simulink model "frequence_response_point3"  (R2019b)
settings: Solver=ode45  StartTime=0.0  StopTime=30  RelTol=1e-3  EnableMultiTasking=on
values from neighbouring files (symbols this model uses):
  C = [1 1 0 0;0 0 1 1]    [es1.m]
  phi = [0 0]    [es1.m]
  U = [1 -0.25]    [es1.m]
  w = [0 2]    [es1.m]
undefined symbols (not defined in the file or in its folder): A, B, D
settings Model: Creator=stefano  LastModifiedBy=Chiara
settings DataIOCC: LimitDataPoints=on  SaveFormat=Array  SignalLoggingSaveFormat=ModelDataLogs  ReturnWorkspaceOutputs=off
settings OptimizationCC: ExpressionDepthLimit=2147483647  LifeSpan=inf
settings DebuggingCC: UnderspecifiedInitializationDetection=Classic  MergeDetectMultiDrivingBlocksExec=none  SolverPrmCheckMsg=warning  FcnCallInpInsideContextMsg=warning  StateNameClashWarn=warning  SFUnexpectedBacktrackingDiag=warning  SFNoUnconditionalDefaultTransitionDiag=warning  SFExecutionAtInitializationDiag=none  ArithmeticOperatorsInVariantConditions=warning
settings HardwareCC: ProdBitPerPointer=32  ProdBitPerSizeT=32  ProdBitPerPtrDiffT=32  ProdLargestAtomicFloat=None  ProdIntDivRoundTo=Undefined  ProdEndianess=Unspecified  ProdWordSize=32  ProdHWDeviceType=32-bit Generic
settings ModelReferenceCC: PropagateSignalLabelsOutOfModel=off
settings SFSimCC: SimUseLocalCustomCode=off  CustomCodeUndefinedFunction=UseInterfaceOnly
settings RTWCC: RTWUseLocalCustomCode=off
settings CodeAppCC: StateflowObjectComments=on
settings GRTTargetCC: TargetLangStandard=C89/C90 (ANSI)  GeneratePreprocessorConditionals=Disable all  CombineOutputUpdateFcns=off  GRTInterface=on
settings ConfigComp: CovMetricSettings=dw  CovHtmlReporting=on  CovSaveCumulativeToWorkspaceVar=on  CovSaveSingleToWorkspaceVar=on  CovExternalEMLEnable=off

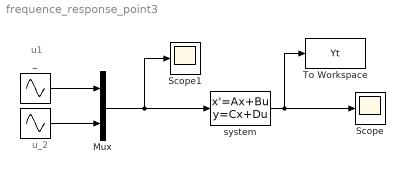
== system frequence_response_point3 ==
  note: u_2
  note: u1
  " " : Sin  Amplitude=U(2)  Frequency=w(2)  Phase=phi(2)  SampleTime=0
  " _" : Sin  Amplitude=U(1)  Frequency=w(1)  Phase=phi(1)  SampleTime=0
  Mux : Mux  Inputs=2
  Scope : Scope
  Scope1 : Scope
  "To Workspace " : ToWorkspace  VariableName=Yt  SaveFormat=Timeseries  SampleTime=-1
  system : StateSpace  A=A  B=B  C=C  D=D  InitialCondition=0
  wires:
  system/1 -> Scope/1, "To Workspace "/1
  Mux/1 -> Scope1/1, system/1
  " "/1 -> Mux/2
  " _"/1 -> Mux/1
